simulink model "hw2"  (R2018b)
settings: Solver=VariableStepAuto  StartTime=0  StopTime=60  RelTol=1e-3
libraries: cstblocks x2
settings Model: Creator=trey  LastModifiedBy=trey

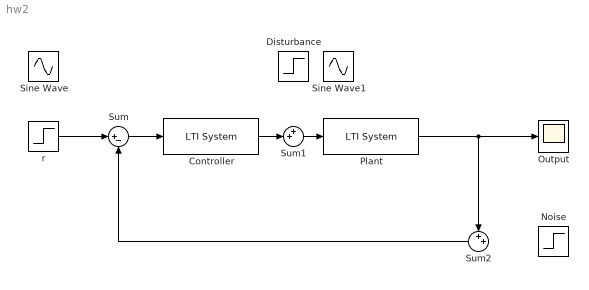
== system hw2 ==
  Controller : cstblocks/LTI System  sys=C  IC=[]
  Disturbance : Step  Time=0  SampleTime=0
  Noise : Step  Time=0  After=3  SampleTime=0
  Output : Scope
  Plant : cstblocks/LTI System  sys=P  IC=[]
  Sine Wave : Sin  Amplitude=2  Frequency=5  SampleTime=0
  Sine Wave1 : Sin  SampleTime=0
  Sum : Sum  Inputs=|+-
  Sum1 : Sum  Inputs=++|
  Sum2 : Sum  Inputs=++|
  r : Step  Time=0  SampleTime=0
  wires:
  Sum1/1 -> Plant/1
  Controller/1 -> Sum1/2
  Plant/1 -> Output/1, Sum2/1
  Sum/1 -> Controller/1
  Sum2/1 -> Sum/2
  r/1 -> Sum/1
